simulink model "inp_const"  (R2023a)
settings: Solver=VariableStepAuto  StartTime=0.0  StopTime=10.0  RelTol=1e-3
settings Model: Creator=Taniya Baral  LastModifiedBy=Taniya Baral

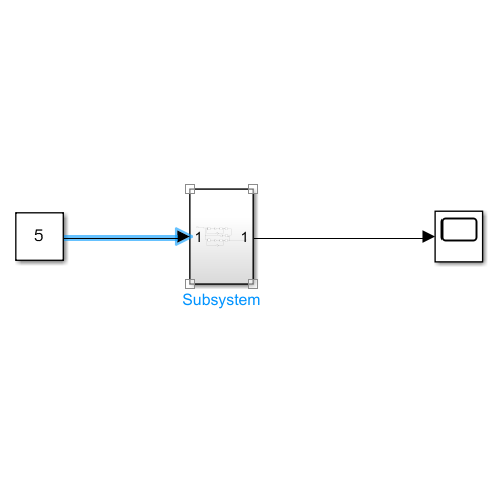
[thumbnail: Simulink's stored preview of the top-level diagram]
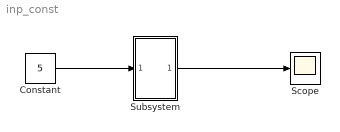
== system inp_const ==
  Constant : Constant  Value=5
  Scope : Scope
  Subsystem : Subsystem
  wires:
  Constant/1 -> Subsystem/1(In1)
  Subsystem/1(Out1) -> Scope/1

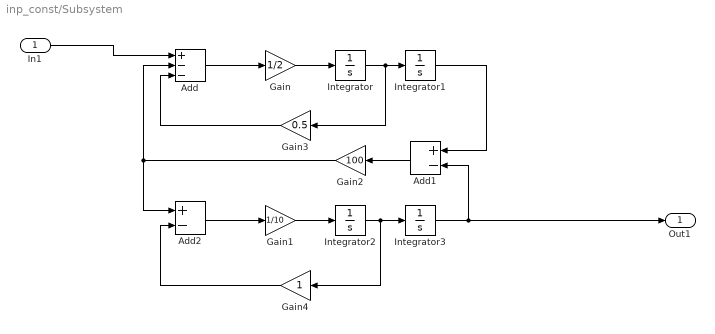
== system inp_const/Subsystem ==
  In1 : Inport
  Add : Sum  Inputs=+--
  Add1 : Sum  Inputs=+-
  Add2 : Sum  Inputs=+-
  Gain : Gain  Gain=1/2
  Gain1 : Gain  Gain=1/10
  Gain2 : Gain  Gain=100
  Gain3 : Gain  Gain=0.5
  Gain4 : Gain
  Integrator{,1..3} (4 alike) : Integrator
  Out1 : Outport
  wires:
  Integrator2/1 -> Gain4/1, Integrator3/1
  Add/1 -> Gain/1
  Gain/1 -> Integrator/1
  Add2/1 -> Gain1/1
  Gain1/1 -> Integrator2/1
  Integrator3/1 -> Out1/1, Add1/2
  Add1/1 -> Gain2/1
  In1/1 -> Add/1
  Integrator/1 -> Gain3/1, Integrator1/1
  Gain2/1 -> Add2/1, Add/2
  Integrator1/1 -> Add1/1
  Gain3/1 -> Add/3
  Gain4/1 -> Add2/2
